simulink model "tp3_exo6"  (R2016a)
settings: Solver=VariableStepAuto  StartTime=0.0  StopTime=200  RelTol=1e-3
values from neighbouring files (symbols this model uses):
  h = (tf-t0)/N    [init.m]    (also in init_tp3.m)
  l = 10    [init.m]    (also in init_TP1.m = 1; init_TP2_controle.m; init_tp3.m = 5)
undefined symbols (not defined in the file or in its folder): DiscIntNeverNeededParam
libraries: simulink x1
settings Model: Creator=plarato  LastModifiedBy=fgaribal

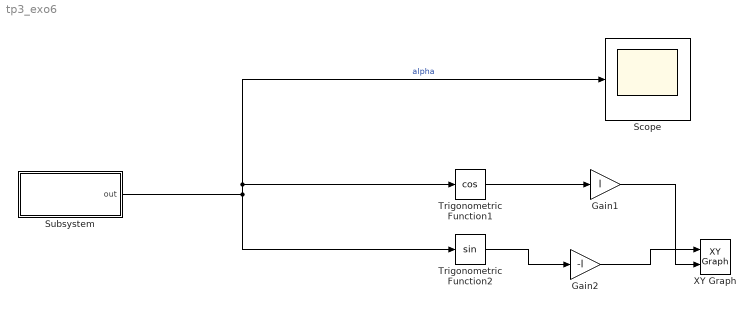
== system tp3_exo6 ==
  Gain1 : Gain  Gain=l
  Gain2 : Gain  Gain=-l
  Scope : Scope
  Subsystem : Subsystem
  Trigonometric Function1 : Trigonometry  Operator=cos
  Trigonometric Function2 : Trigonometry
  XY Graph : simulink/Sinks/XY Graph  xmin=-l  xmax=l  ymin=-l  ymax=l  st=-1
  wires:
  Trigonometric Function1/1 -> Gain1/1
  Trigonometric Function2/1 -> Gain2/1
  Gain2/1 -> XY Graph/1
  Gain1/1 -> XY Graph/2
  Subsystem/1("out ") -> Trigonometric Function2/1, Scope/1, Trigonometric Function1/1  "alpha"

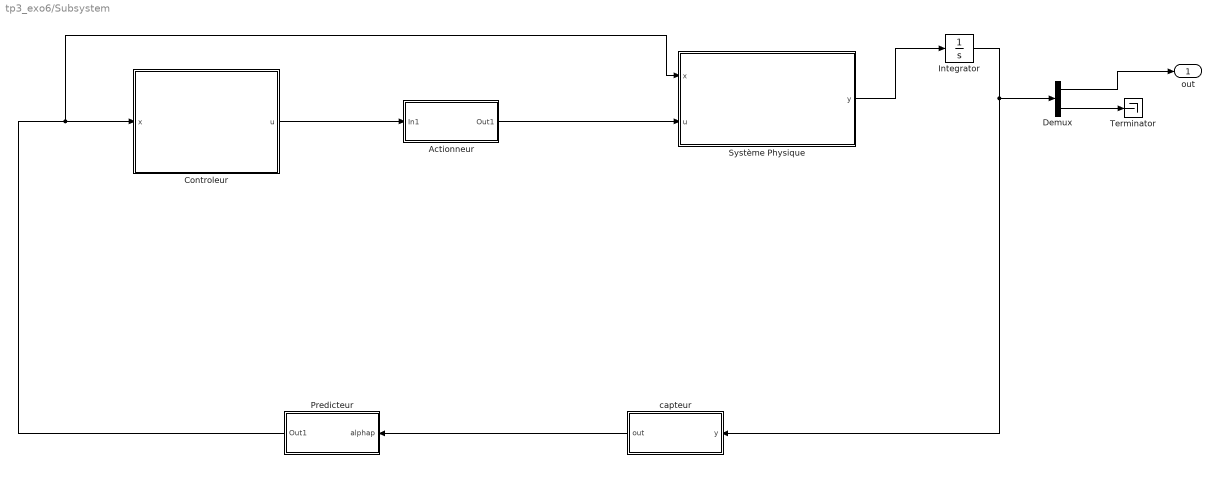
== system tp3_exo6/Subsystem ==
  Actionneur : Subsystem
  Controleur : Subsystem
  Demux : Demux  Outputs=2
  Integrator : Integrator  InitialCondition=pi/4
  Predicteur : Subsystem
  "Système Physique " : Subsystem
  Terminator : Terminator
  "capteur " : Subsystem
  "out " : Outport
  wires:
  "capteur "/1(out) -> Predicteur/1(alphap)
  Controleur/1(u) -> Actionneur/1(In1)
  Actionneur/1(Out1) -> "Système Physique "/2(u)
  Integrator/1 -> "capteur "/1(y), Demux/1
  Demux/1 -> "out "/1
  Demux/2 -> Terminator/1
  Predicteur/1(Out1) -> "Système Physique "/1(x), Controleur/1(x)
  "Système Physique "/1("y ") -> Integrator/1

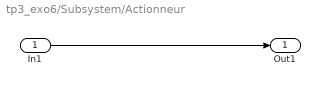
== system tp3_exo6/Subsystem/Actionneur ==
  In1 : Inport
  Out1 : Outport
  wires:
  In1/1 -> Out1/1

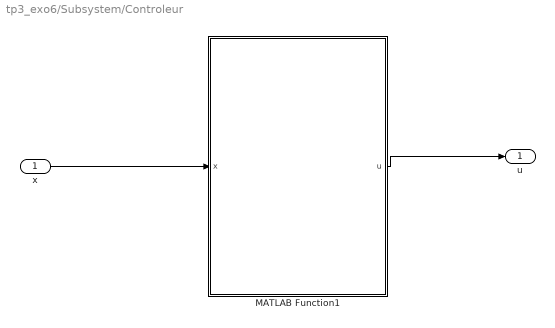
== system tp3_exo6/Subsystem/Controleur ==
  x : Inport
  MATLAB Function1 : MATLAB Function  TreatAsAtomicUnit=on
  u : Outport
  wires:
  MATLAB Function1/1(u) -> u/1
  x/1 -> MATLAB Function1/1(x)

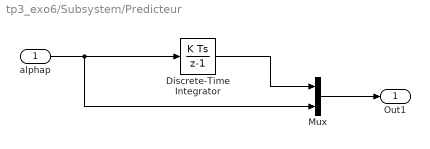
== system tp3_exo6/Subsystem/Predicteur ==
  alphap : Inport
  Discrete-Time Integrator : DiscreteIntegrator  InitialConditionSetting=State (most efficient)  SampleTime=25*h  ICPrevOutput=DiscIntNeverNeededParam  ICPrevScaledInput=DiscIntNeverNeededParam
  Mux : Mux  Inputs=2
  Out1 : Outport
  wires:
  alphap/1 -> Discrete-Time Integrator/1, Mux/2
  Mux/1 -> Out1/1
  Discrete-Time Integrator/1 -> Mux/1

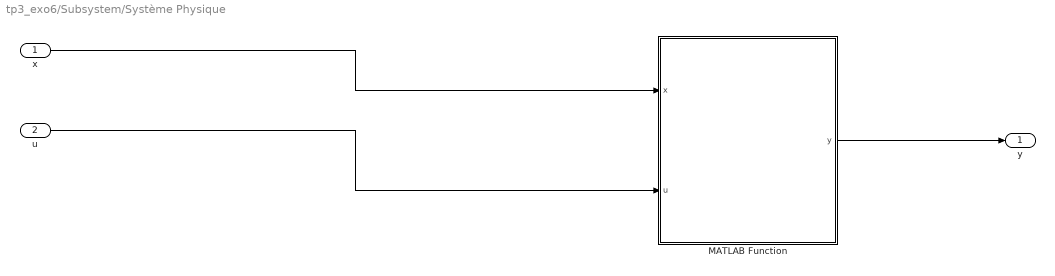
== system tp3_exo6/Subsystem/Système Physique  ==
  x : Inport
  u : Inport  Port=2
  MATLAB Function : MATLAB Function  TreatAsAtomicUnit=on
  "y " : Outport
  wires:
  MATLAB Function/1(y) -> "y "/1
  u/1 -> MATLAB Function/2(u)
  x/1 -> MATLAB Function/1(x)

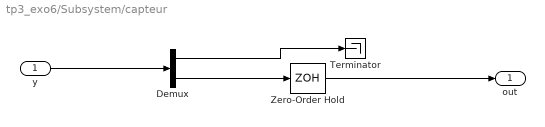
== system tp3_exo6/Subsystem/capteur  ==
  y : Inport
  Demux : Demux  Outputs=2
  Terminator : Terminator
  Zero-Order Hold : ZeroOrderHold  SampleTime=25*h
  out : Outport
  wires:
  Demux/1 -> Terminator/1
  y/1 -> Demux/1
  Demux/2 -> Zero-Order Hold/1
  Zero-Order Hold/1 -> out/1

== matlab function tp3_exo6/Subsystem/Controleur/MATLAB Function1 ==
  data: x input; u output
%Controleur
function u = fcn(x)
%#codegen
ue=0;
K=[20;10];
xe = [0;0];

u = ue + K'*(x - xe);

== matlab function tp3_exo6/Subsystem/Système Physique /MATLAB Function ==
  data: x input; y output; u input
function y = fcn(x,u)
%#codegen
g=9.81;
l=10;
y = zeros(2,1);
y(1) = x(2);
y(2) = (g/l)*sin(x(1))-(u*cos(x(1))/l);
